simulink model "SistemaLineal"  (R2018b)
settings: Solver=VariableStepAuto  StartTime=0.0  StopTime=ttotal  RelTol=1e-3
values from neighbouring files (symbols this model uses):
  denom = [1 -0.2 0.5 -0.1]    [Prueba.m]
  denom2 = [1 -.5 .04]    [Otra_prueba_mas.m]    (also in Prueba.m = [1 -0.3 0.4 0.5])
  iseed = randi(2^53-1)    [IdentificacionTS.m]    (also in Otra_prueba_mas.m = randi(5000))
  num = [0 0 1 0.2]    [Prueba.m]
  num2 = [0 2 -.6]    [Otra_prueba_mas.m]    (also in Prueba.m = [0 0 0 1])
  tmuestra = 0.05    [ControlDeEstadosTS.m]    (also in IdentificacionTS.m; Otra_prueba_mas.m; Prueba.m)
  var = 0.001    [IdentificacionTS.m]    (also in Prueba.m = 1e-05)
settings Model: Creator=pablo  LastModifiedBy=pablo

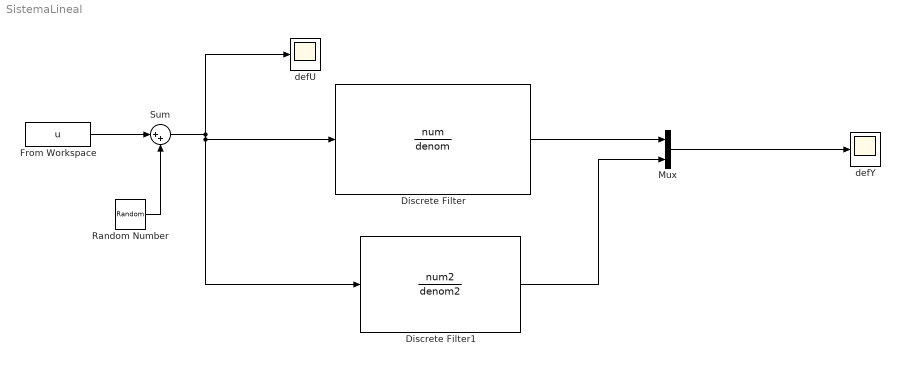
== system SistemaLineal ==
  Discrete Filter : DiscreteFilter  Numerator=num  Denominator=denom
  Discrete Filter1 : DiscreteFilter  Numerator=num2  Denominator=denom2
  From Workspace : FromWorkspace  VariableName=u  SampleTime=tmuestra
  Mux : Mux  Inputs=2
  Random Number : RandomNumber  Variance=var  Seed=iseed  SampleTime=tmuestra
  Sum : Sum  Inputs=|++
  "defU " : Scope
  "defY " : Scope
  wires:
  From Workspace/1 -> Sum/1
  Random Number/1 -> Sum/2
  Sum/1 -> Discrete Filter1/1, Discrete Filter/1, "defU "/1
  Discrete Filter/1 -> Mux/1
  Discrete Filter1/1 -> Mux/2
  Mux/1 -> "defY "/1
